simulink model "Control_model_matching_no_lineal"  (R2023a)
settings: Solver=FixedStepAuto  StartTime=0.0  StopTime=70  FixedStep=Ts  RelTol=1e-3
values from neighbouring files (symbols this model uses):
  IMU1_aB = [0.000820278190076 0.00115353439469 0.000894968456123]    [DatosSimulador.mat]
  IMU1_aK = [1.26449540403e-05 4.27040286013e-05 5.33261409146e-05]    [DatosSimulador.mat]
  IMU1_aN = [0.00684624677524 0.00597589835525 0.00590605800971]    [DatosSimulador.mat]
  IMU1_gB = [0.000430438056355 0.000168108439539 0.000519584631547]    [DatosSimulador.mat]
  IMU1_gK = [3.54504736606e-05 3.3319713566e-06 4.94506384712e-05]    [DatosSimulador.mat]
  IMU1_gN = [0.0047084921971 0.00506619736552 0.00340488785878]    [DatosSimulador.mat]
  IMU2_aB = [0.00173700635787 0.00079356651986 0.000918277248275]    [DatosSimulador.mat]
  IMU2_aK = [0.000253509817412 2.45614519372e-05 6.68535212753e-05]    [DatosSimulador.mat]
  IMU2_aN = [0.00535466242582 0.00533867441118 0.00558323645964]    [DatosSimulador.mat]
  IMU2_gB = [0.000335599994287 0.000795064377598 0.00045980210416]    [DatosSimulador.mat]
  IMU2_gK = [3.18091115332e-05 5.54514226678e-05 3.22930100083e-05]    [DatosSimulador.mat]
  IMU2_gN = [0.00695891398937 0.00398353487253 0.00368572026491]    [DatosSimulador.mat]
  IMU3_aB = [0.000325683271512 0.000441587151727 0.000601047067903]    [DatosSimulador.mat]
  IMU3_aK = [1.00979314084e-05 2.18555360334e-05 3.5534689232e-05]    [DatosSimulador.mat]
  IMU3_aN = [0.00413628574461 0.00448110466823 0.00368606415577]    [DatosSimulador.mat]
  IMU3_gB = [0.000501559406985 0.000889874761924 0.000218087094254]    [DatosSimulador.mat]
  IMU3_gK = [1.959913061e-05 4.03655103582e-05 4.44406532552e-06]    [DatosSimulador.mat]
  IMU3_gN = [0.00573350535706 0.0096154846251 0.00568739091977]    [DatosSimulador.mat]
  Ts = 0.001    [DatosSimulador.mat]
  TsMot = 0.001    [DatosSimulador.mat]
  TsPos = 0.002    [DatosSimulador.mat]
  TsRef = 0.02    [DatosSimulador.mat]
  TsSenB = 0.001    [DatosSimulador.mat]
  TsSenF = 0.001    [DatosSimulador.mat]
  TsVel = 0.001    [DatosSimulador.mat]
undefined symbols (not defined in the file or in its folder): denG, denM, numG, numM
libraries: mspsensorlib x3, simulink x2
(part 3 of 3)

== matlab function Control_model_matching_no_lineal/Estimacion/IMU 1/Filtro pasa bajos giroscopio/MATLAB Function1 ==
  settings: updateMethod=DISCRETE
  data: In input; Fc input; Out output; Ts input
function Out  = LowPassFilterP2(In, Fc, Ts)

persistent b0 b1 b2 a1 a2 a0 in1 in2 out1 out2

if isempty(b0)
    ohm     = 2 * pi * Fc;
    damping = 1 / (sqrt(2));

    b2 = Ts^2 * ohm^2;
    b1 = 2.0 * b2;
    b0 = b2;

    a2 = 4.0 + 4.0 * damping * ohm * Ts + b2;
    a1 = -8.0 + b1;
    a0 = 4.0 - 4.0 * damping * ohm * Ts + b2;

    in1  = 0;
    in2  = 0;
    out1 = 0;
    out2 = 0;
end

Out = (b2 * In + b1 * in1 + b0 * in2 - a1 * out1 - a0 * out2) / a2;

in2  = in1;
in1  = In;
out2 = out1;
out1 = Out;

== matlab function Control_model_matching_no_lineal/Estimacion/IMU 1/Filtro pasa bajos giroscopio/MATLAB Function2 ==
  settings: updateMethod=DISCRETE
  data: In input; Fc input; Out output; Ts input
function Out  = LowPassFilterP2(In, Fc, Ts)

persistent b0 b1 b2 a1 a2 a0 in1 in2 out1 out2

if isempty(b0)
    ohm     = 2 * pi * Fc;
    damping = 1 / (sqrt(2));

    b2 = Ts^2 * ohm^2;
    b1 = 2.0 * b2;
    b0 = b2;

    a2 = 4.0 + 4.0 * damping * ohm * Ts + b2;
    a1 = -8.0 + b1;
    a0 = 4.0 - 4.0 * damping * ohm * Ts + b2;

    in1  = 0;
    in2  = 0;
    out1 = 0;
    out2 = 0;
end

Out = (b2 * In + b1 * in1 + b0 * in2 - a1 * out1 - a0 * out2) / a2;

in2  = in1;
in1  = In;
out2 = out1;
out1 = Out;

== matlab function Control_model_matching_no_lineal/Estimacion/IMU 1/Filtro pasa bajos giroscopio/MATLAB Function3 ==
  settings: updateMethod=DISCRETE
  data: In input; Fc input; Out output; Ts input
function Out  = LowPassFilterP1(In, Fc, Ts)

persistent b0 b1 a0 a1 in1 out1

if isempty(b0)
    ohm = 2.0 * pi * Fc;

    b1 = ohm * Ts;
    b0 = b1;
    a1 = 2.0 + b1;
    a0 = b1 - 2.0;

    in1  = 0;
    out1 = 0;
end

Out = (b1 * In + b0 * in1 - a0 * out1) / a1;

in1  = In;
out1 = Out;

== matlab function Control_model_matching_no_lineal/Estimacion/IMU 1/Filtro pasa bajos giroscopio/MATLAB Function4 ==
  settings: updateMethod=DISCRETE
  data: In input; Fc input; Out output; Ts input
function Out  = LowPassFilterP1(In, Fc, Ts)

persistent b0 b1 a0 a1 in1 out1

if isempty(b0)
    ohm = 2.0 * pi * Fc;

    b1 = ohm * Ts;
    b0 = b1;
    a1 = 2.0 + b1;
    a0 = b1 - 2.0;

    in1  = 0;
    out1 = 0;
end

Out = (b1 * In + b0 * in1 - a0 * out1) / a1;

in1  = In;
out1 = Out;

== matlab function Control_model_matching_no_lineal/Estimacion/IMU 1/Filtro pasa bajos giroscopio/MATLAB Function5 ==
  settings: updateMethod=DISCRETE
  data: In input; Fc input; Out output; Ts input
function Out  = LowPassFilterP2(In, Fc, Ts)

persistent b0 b1 b2 a1 a2 a0 in1 in2 out1 out2

if isempty(b0)
    ohm     = 2 * pi * Fc;
    damping = 1 / (sqrt(2));

    b2 = Ts^2 * ohm^2;
    b1 = 2.0 * b2;
    b0 = b2;

    a2 = 4.0 + 4.0 * damping * ohm * Ts + b2;
    a1 = -8.0 + b1;
    a0 = 4.0 - 4.0 * damping * ohm * Ts + b2;

    in1  = 0;
    in2  = 0;
    out1 = 0;
    out2 = 0;
end

Out = (b2 * In + b1 * in1 + b0 * in2 - a1 * out1 - a0 * out2) / a2;

in2  = in1;
in1  = In;
out2 = out1;
out1 = Out;

== matlab function Control_model_matching_no_lineal/Estimacion/IMU 1/Filtro pasa bajos giroscopio/MATLAB Function6 ==
  settings: updateMethod=DISCRETE
  data: In input; Fc input; Out output; Ts input
function Out  = LowPassFilterP1(In, Fc, Ts)

persistent b0 b1 a0 a1 in1 out1

if isempty(b0)
    ohm = 2.0 * pi * Fc;

    b1 = ohm * Ts;
    b0 = b1;
    a1 = 2.0 + b1;
    a0 = b1 - 2.0;

    in1  = 0;
    out1 = 0;
end

Out = (b1 * In + b0 * in1 - a0 * out1) / a1;

in1  = In;
out1 = Out;

== matlab function Control_model_matching_no_lineal/Estimacion/IMU 1/Sensor IMU/MATLAB Function5 ==
  data: Wb input; Q input; Vel output
function Vel = RotacionVelBT(Wb, Q)

Euler = [0 0 0]';

Euler(1) = atan2(2 * Q(3) * Q(4) + 2 * Q(1) * Q(2), 2 * Q(1) * Q(1) + 2 * Q(4) * Q(4) - 1);
Euler(2) = -asin(2 * (Q(2) * Q(4) - Q(1) * Q(3)));
Euler(3) = atan2(2 * Q(2) * Q(3) + 2 * Q(1) * Q(4), 2 * Q(1) * Q(1) + 2 * Q(2) * Q(2) - 1);


w1 = Wb(1) + Wb(2) * sin(Euler(1)) * tan(Euler(2)) + Wb(3) * cos(Euler(1)) * tan(Euler(2));
w2 = Wb(2) * cos(Euler(1)) - Wb(3) * sin(Euler(1));
w3 = Wb(2) * sin(Euler(1)) / cos(Euler(2)) + Wb(3) * cos(Euler(1)) / cos(Euler(2));

Vel = [w1 w2 w3];

== matlab function Control_model_matching_no_lineal/Estimacion/MATLAB Function ==
  data: Euler input; Wb input; Vel output
function Vel = RotacionVelBT(Euler, Wb)

w1 = Wb(1) + Wb(2) * sin(Euler(1)) * tan(Euler(2)) + Wb(3) * cos(Euler(1)) * tan(Euler(2));
w2 = Wb(2) * cos(Euler(1)) - Wb(3) * sin(Euler(1));
w3 = Wb(2) * sin(Euler(1)) / cos(Euler(2)) + Wb(3) * cos(Euler(1)) / cos(Euler(2));

Vel = [w1 w2 w3];

== matlab function Control_model_matching_no_lineal/Estimacion/IMU 1/MATLAB Function1 ==
  data: u input; max input; acumW1 data_store_memory; cntW1 data_store_memory
function escribirAcumuladorW(u, max)

global acumW1 cntW1

acumW1 = acumW1 + u;
cntW1  = cntW1 + 1;

if cntW1 >= max
    cntW1 = max / 2;
    acumW1 = acumW1 / 2;
end

== matlab function Control_model_matching_no_lineal/Estimacion/IMU 1/MATLAB Function2 ==
  data: y output; acumW1 data_store_memory; cntW1 data_store_memory
function y = leerAcumuladorW

global acumW1 cntW1
persistent valor

if isempty(valor)
    valor = [0 0 0]';
end

if cntW1 ~= 0
    valor = acumW1 / cntW1;
    acumW1 = [0 0 0]';
    cntW1  = 0;
end
    
y = valor;

== matlab function Control_model_matching_no_lineal/Estimacion/IMU 1/MATLAB Function3 ==
  data: y output; acumA1 data_store_memory; cntA1 data_store_memory
function y = leerAcumuladorA

global acumA1 cntA1
persistent valor

if isempty(valor)
    valor = [0 0 0]';
end

if cntA1 ~= 0
    valor  = acumA1 / cntA1;
    acumA1 = [0 0 0]';
    cntA1  = 0;
end

y = valor;

== matlab function Control_model_matching_no_lineal/Estimacion/IMU 1/MATLAB Function4 ==
  data: u input; max input; acumA1 data_store_memory; cntA1 data_store_memory
function escribirAcumuladorA(u, max)

global acumA1 cntA1

acumA1 = acumA1 + u;
cntA1  = cntA1 + 1;

if cntA1 >= max
    cntA1 = max / 2;
    acumA1 = acumA1 / 2;
end

== matlab function Control_model_matching_no_lineal/Estimacion/IMU 3/Filtro pasa bajos giroscopio/MATLAB Function6 ==
  settings: updateMethod=DISCRETE
  data: In input; Fc input; Out output; Ts input
function Out  = LowPassFilterP1(In, Fc, Ts)

persistent b0 b1 a0 a1 in1 out1

if isempty(b0)
    ohm = 2.0 * pi * Fc;

    b1 = ohm * Ts;
    b0 = b1;
    a1 = 2.0 + b1;
    a0 = b1 - 2.0;

    in1  = 0;
    out1 = 0;
end

Out = (b1 * In + b0 * in1 - a0 * out1) / a1;

in1  = In;
out1 = Out;

== matlab function Control_model_matching_no_lineal/Estimacion/AHRS/MATLAB Function ==
  data: zeta input; beta input; gir input; acel input; tiempo input; Q output
function Q = Madgwick(zeta, beta, gir, acel, tiempo)

persistent tiempoAnterior q bias

if isempty(q)
    tiempoAnterior = 0;
    q    = [1 0 0 0]';
    bias = [0 0 0]';
end

qDot = [0 0 0 0]';
s    = [0 0 0 0]';
e    = [0 0 0]';
vel  = [0 0 0]';

dt = tiempo - tiempoAnterior;
tiempoAnterior = tiempo;

if (~((acel(1) == 0) && (acel(2) == 0) && (acel(3) == 0))) 

	% Se normaliza la acelereacion
    normA = norm(acel);
    if normA ~= 0 
        a = acel / normA;
    else
        a = acel;
    end

    % Variables auxiliares del cuaternion
    q2_1 = 2.0 * q(1);
    q2_2 = 2.0 * q(2);
    q2_3 = 2.0 * q(3);
    q2_4 = 2.0 * q(4);
    q4_1 = 4.0 * q(1);
    q4_2 = 4.0 * q(2);
    q4_3 = 4.0 * q(3);
    q8_2 = 8.0 * q(2);
    q8_3 = 8.0 * q(3);
    q1q1 = q(1) * q(1);
    q2q2 = q(2) * q(2);
    q3q3 = q(3) * q(3);
    q4q4 = q(4) * q(4);

    % Correccion del algoritmo
    s(1) = q4_1 * q3q3 + q2_3 * a(1) + q4_1 * q2q2 - q2_2 * a(2);
    s(2) = q4_2 * q4q4 - q2_4 * a(1) + 4.0  * q1q1 * q(2) - q2_1 * a(2) - q4_2 + q8_2 * q2q2 + q8_2 * q3q3 + q4_2 * a(3);
    s(3) = 4.0  * q1q1 * q(3) + q2_1 * a(1) + q4_3 * q4q4 - q2_4 * a(2) - q4_3 + q8_3 * q2q2 + q8_3 * q3q3 + q4_3 * a(3);
    s(4) = 4.0  * q2q2 * q(4) - q2_2 * a(1) + 4.0 * q3q3 * q(4) - q2_3 * a(2);

    normS = norm(s);
    if normS ~= 0 
        s = s / normS;
    end

    % Compensacion del bias
    e(1) = 2 * q(1) * s(2) - 2 * q(2) * s(1) - 2 * q(3) * s(4) + 2 * q(4) * s(3);
    e(2) = 2 * q(1) * s(3) + 2 * q(2) * s(4) - 2 * q(3) * s(1) - 2 * q(4) * s(2);
    e(3) = 2 * q(1) * s(4) - 2 * q(2) * s(3) + 2 * q(3) * s(2) - 2 * q(4) * s(1);

    bias(1) = bias(1) + e(1) * dt * zeta;
    bias(2) = bias(2) + e(2) * dt * zeta;
    bias(3) = bias(3) + e(3) * dt * zeta;

    vel(1) = gir(1) - bias(1);
    vel(2) = gir(2) - bias(2);
    vel(3) = gir(3) - bias(3);

	% Tasa de cambio del cuaternion
    qDot(1) = 0.5 * (-q(2) * vel(1) - q(3) * vel(2) - q(4) * vel(3));
    qDot(2) = 0.5 * ( q(1) * vel(1) + q(3) * vel(3) - q(4) * vel(2));
    qDot(3) = 0.5 * ( q(1) * vel(2) - q(2) * vel(3) + q(4) * vel(1));
    qDot(4) = 0.5 * ( q(1) * vel(3) + q(2) * vel(2) - q(3) * vel(1));

    % Se aplica el feedback
    qDot(1) = qDot(1) - beta * s(1);
    qDot(2) = qDot(2) - beta * s(2);
    qDot(3) = qDot(3) - beta * s(3);
    qDot(4) = qDot(4) - beta * s(4);
end

% Se integra el cuaternion
q(1) = q(1) + qDot(1) * dt;
q(2) = q(2) + qDot(2) * dt;
q(3) = q(3) + qDot(3) * dt;
q(4) = q(4) + qDot(4) * dt;

% Se normaliza el cuaternion
Q = q / norm(q);

== matlab function Control_model_matching_no_lineal/Estimacion/IMU 3/MATLAB Function1 ==
  data: u input; max input; acumW3 data_store_memory; cntW3 data_store_memory
function escribirAcumuladorW(u, max)

global acumW3 cntW3

acumW3 = acumW3 + u;
cntW3  = cntW3 + 1;

if cntW3 >= max
    cntW3  = max / 2;
    acumW3 = acumW3 / 2;
end

== matlab function Control_model_matching_no_lineal/Estimacion/IMU 3/MATLAB Function2 ==
  data: y output; acumW3 data_store_memory; cntW3 data_store_memory
function y = leerAcumuladorW

global acumW3 cntW3
persistent valor

if isempty(valor)
    valor = [0 0 0]';
end

if cntW3 ~= 0
    valor  = acumW3 / cntW3;
    acumW3 = [0 0 0]';
    cntW3  = 0;
end
    
y = valor;

== matlab function Control_model_matching_no_lineal/Estimacion/IMU 3/MATLAB Function3 ==
  data: y output; acumA3 data_store_memory; cntA3 data_store_memory
function y = leerAcumuladorA

global acumA3 cntA3
persistent valor

if isempty(valor)
    valor = [0 0 0]';
end

if cntA3 ~= 0
    valor  = acumA3 / cntA3;
    acumA3 = [0 0 0]';
    cntA3  = 0;
end

y = valor;

== matlab function Control_model_matching_no_lineal/Estimacion/IMU 3/MATLAB Function4 ==
  data: u input; max input; acumA3 data_store_memory; cntA3 data_store_memory
function escribirAcumuladorA(u, max)

global acumA3 cntA3

acumA3 = acumA3 + u;
cntA3  = cntA3 + 1;

if cntA3 >= max
    cntA3  = max / 2;
    acumA3 = acumA3 / 2;
end

== matlab function Control_model_matching_no_lineal/Estimacion/IMU 3/Sensor IMU/MATLAB Function5 ==
  data: Wb input; Q input; Vel output
function Vel = RotacionVelBT(Wb, Q)

Euler = [0 0 0]';

Euler(1) = atan2(2 * Q(3) * Q(4) + 2 * Q(1) * Q(2), 2 * Q(1) * Q(1) + 2 * Q(4) * Q(4) - 1);
Euler(2) = -asin(2 * (Q(2) * Q(4) - Q(1) * Q(3)));
Euler(3) = atan2(2 * Q(2) * Q(3) + 2 * Q(1) * Q(4), 2 * Q(1) * Q(1) + 2 * Q(2) * Q(2) - 1);


w1 = Wb(1) + Wb(2) * sin(Euler(1)) * tan(Euler(2)) + Wb(3) * cos(Euler(1)) * tan(Euler(2));
w2 = Wb(2) * cos(Euler(1)) - Wb(3) * sin(Euler(1));
w3 = Wb(2) * sin(Euler(1)) / cos(Euler(2)) + Wb(3) * cos(Euler(1)) / cos(Euler(2));

Vel = [w1 w2 w3];

== matlab function Control_model_matching_no_lineal/Modelo UAV/Dinamica UAV/Modelo ==
  settings: updateMethod=DISCRETE
  data: Ab output; T input; Delta input; Wm input; Gb output; I input; Im input; B input; F input; dM input; M input; Dr input; Dp input; Mo input; HabYaw input; HabAcel input; Wb input size=3; Velb input size=3; Q input size=4; Tiempo input; Al output
function [Ab, Gb, Al] = Modelo(T, Delta, Wm, I, Im, B, F, dM, M, Dr, Dp, Mo, HabYaw, HabAcel, Wb, Velb, Q, Tiempo)
% Modelo matemático del UAV 

%%%%%%%%%%%%%%%%%%%%%%%%%%%%%%% ENTRADAS %%%%%%%%%%%%%%%%%%%%%%%%%%%%%%%%%%%%%%%%%%%%%%%%%%
% T     -> Fuerza de sustentación
% Delta -> Par de arraste 
% Wm    -> Velocidad de rotacion de los rotores
% I     -> Inercia del dron
% Im    -> Inercia del rotor
% B     -> Friccion viscosa
% F     -> Friccion estatica
% dM    -> Distancia al centro de masas
% M     -> Masa del dron
% Dr    -> Distancia al eje roll
% Dp    -> Distancia al eje pitch
% Mo    -> Par inicial
% HabYaw -> Habilitacion de yaw
% HabAcel
% Wb    -> Velocidades angulares en el cuerpo
% Euler -> Angulos de Euler


%%%%%%%%%%%%%%%%%%%%%%%%%%%%%%% SALIDAS %%%%%%%%%%%%%%%%%%%%%%%%%%%%%%%%%%%%%%%%%%%%%%%%%%%
% Ab  -> Aceleración angular en los 3 ejes
% Gb  -> Gravedad en el sistema de referencia del dron


%%%%%%%%%%%%%%%%%%%%%%%%%%%%% CONSTANTES %%%%%%%%%%%%%%%%%%%%%%%%%%%%%%%%%%%%%%%%%%%%%%%%%%
persistent g LrAnt TiempoAnterior

if isempty(g)
    g = 9.81;
    LrAnt = 0;
    TiempoAnterior = 0;
end


%%%%%%%%%%%%%%%%%%%%%%%%%%%%%% VARIABLES %%%%%%%%%%%%%%%%%%%%%%%%%%%%%%%%%%%%%%%%%%%%%%%%%%
Fe = zeros(1,3);
Euler = zeros(1,3);

dt = Tiempo - TiempoAnterior;
TiempoAnterior = Tiempo;


%%%%%%%%%%%%%%%%%%%%%%%%% ANGULOS Y ROTACIONES %%%%%%%%%%%%%%%%%%%%%%%%%%%%%%%%%%%%%%%%%%%%
% Angulos de Euler
Euler(1) = atan2(2 * Q(3) * Q(4) + 2 * Q(1) * Q(2), 2 * Q(1) * Q(1) + 2 * Q(4) * Q(4) - 1);
Euler(2) = -asin(2 * (Q(2) * Q(4) - Q(1) * Q(3)));
Euler(3) = atan2(2 * Q(2) * Q(3) + 2 * Q(1) * Q(4), 2 * Q(1) * Q(1) + 2 * Q(2) * Q(2) - 1);

% Matriz de rotación
R = [[1-2*Q(3)^2-2*Q(4)^2 2*(Q(2)*Q(3)+Q(1)*Q(4)) 2*(Q(2)*Q(4)-Q(1)*Q(3))];...
    [2*(Q(2)*Q(3)-Q(1)*Q(4)) 1-2*Q(2)^2-2*Q(4)^2 2*(Q(3)*Q(4)+Q(1)*Q(2))];...
    [2*(Q(2)*Q(4)+Q(1)*Q(3)) 2*(Q(3)*Q(4)-Q(1)*Q(2)) 1-2*Q(2)^2-2*Q(3)^2]];


%%%%%%%%%%%%%%%%%%%%%%%%%%% DINAMICA ANGULAR %%%%%%%%%%%%%%%%%%%%%%%%%%%%%%%%%%%%%%%%%%%%%%
% Pares generados por los rotores
Mx = Dr * (T(2) + T(3) - T(1) - T(4));              
My = Dp * (T(1) + T(2) - T(3) - T(4));               
Mz = Delta(1) - Delta(2) + Delta(3) - Delta(4); 

% Calculo de inercia de la masa rotante de los motores
Lr  = Im * (- Wm(1) + Wm(2) - Wm(3) + Wm(4));
ALr = (Lr - LrAnt) / dt;
LrAnt = Lr;

% Fricción estatica
Fe(1) = sign(Wb(1)) * F(1);
Fe(2) = sign(Wb(2)) * F(2);
Fe(3) = sign(Wb(3)) * F(3);

% Momentos en la aeronave
Tx = Mx + (I(2) - I(3)) * Wb(2) * Wb(3) - Lr * Wb(2) - B(1) * Wb(1) - Fe(1) + Mo(1) - M * g * dM * sin(Euler(1));
Ty = My + (I(3) - I(1)) * Wb(1) * Wb(3) - Lr * Wb(1) - B(2) * Wb(2) - Fe(2) + Mo(2) - M * g * dM * cos(Euler(1)) * sin(Euler(2));

if HabYaw
    Tz = Mz + Wb(1) * I(1) * 2 + Wb(2) * I(2) + ALr  - B(3) * Wb(3) - Fe(3) + Mo(3);
else
    Tz = 0;
end

% Obtención de la aceleracion angular
Ax = Tx / I(1);
Ay = Ty / I(2);
Az = Tz / I(3);

Ab = [Ax Ay Az]';


%%%%%%%%%%%%%%%%%%%%%%%%%%% DINAMICA LINEAL %%%%%%%%%%%%%%%%%%%%%%%%%%%%%%%%%%%%%%%%%%%%%%%
% Gravedad con respecto al body
Gb = R * [0 0 1]';

% Aceleraciones lineales
if HabAcel
    AcelX = Gb(1) * g + Wb(3) * Velb(2) - Wb(2) * Velb(3);                                                 
    AcelY = Gb(2) * g + Wb(1) * Velb(3) - Wb(3) * Velb(1);                                                 
    AcelZ = Gb(3) * g + Wb(2) * Velb(1) - Wb(1) * Velb(2) - (T(1) + T(2) + T(3) + T(4)) / M;
    
    Al = [AcelX AcelY AcelZ]';
else
    Al = [0 0 0]';
end
